simulink model "suspmod_yime_response"  (R2014a)
settings: Solver=ode45  SolverMode=SingleTasking  StartTime=0.0  StopTime=50  RelTol=1e-3  AbsTol=1e-6
settings Model: Creator=Rick  LastModifiedBy=JATIN
settings DataIOCC: LimitDataPoints=off  SignalLoggingSaveFormat=ModelDataLogs
settings OptimizationCC: BlockReduction=off  BooleanDataType=off  ExpressionDepthLimit=2147483647
settings DebuggingCC: SaveWithParameterizedLinksMsg=none  UnderspecifiedInitializationDetection=Classic  SignalResolutionControl=TryResolveAllWithWarning  SolverPrmCheckMsg=none  InheritedTsInSrcMsg=none  MultiTaskDSMMsg=warning  MultiTaskCondExecSysMsg=none  FcnCallInpInsideContextMsg=EnableAllAsWarning  UnknownTsInhSupMsg=none  StateNameClashWarn=warning
settings HardwareCC: TargetUnknown=on
settings RTWCC: IncludeERTFirstTime=on

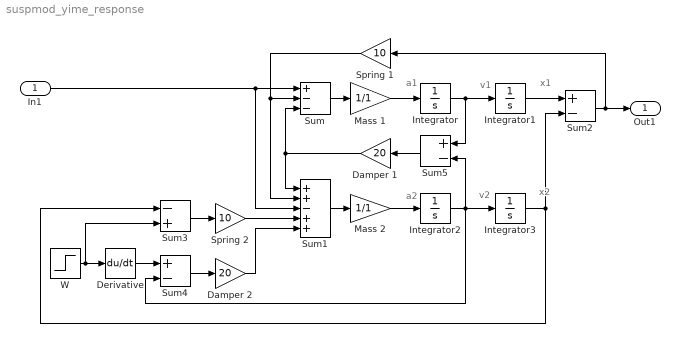
== system suspmod_yime_response ==
  note: a1
  note: v1
  note: x1
  note: a2
  note: v2
  note: x2
  In1 : Inport
  Damper 1 : Gain  Gain=20  SaturateOnIntegerOverflow=on  OutDataTypeStr=Inherit: Same as input  ParamDataTypeStr=Inherit: Same as input
  Damper 2 : Gain  Gain=20  SaturateOnIntegerOverflow=on  OutDataTypeStr=Inherit: Same as input  ParamDataTypeStr=Inherit: Same as input
  Derivative : Derivative
  Integrator{,1..3} (4 alike) : Integrator
  Mass 1 : Gain  Gain=1/1  SaturateOnIntegerOverflow=on  OutDataTypeStr=Inherit: Same as input  ParamDataTypeStr=Inherit: Same as input
  Mass 2 : Gain  Gain=1/1  SaturateOnIntegerOverflow=on  OutDataTypeStr=Inherit: Same as input  ParamDataTypeStr=Inherit: Same as input
  Spring 1 : Gain  Gain=10  SaturateOnIntegerOverflow=on  OutDataTypeStr=Inherit: Same as input  ParamDataTypeStr=Inherit: Same as input
  Spring 2 : Gain  Gain=10  SaturateOnIntegerOverflow=on  OutDataTypeStr=Inherit: Same as input  ParamDataTypeStr=Inherit: Same as input
  Sum : Sum  Inputs=+--  SaturateOnIntegerOverflow=on  InputSameDT=on  OutDataTypeStr=Inherit: Same as first input
  Sum1 : Sum  Inputs=++-++  SaturateOnIntegerOverflow=on  InputSameDT=on  OutDataTypeStr=Inherit: Same as first input
  Sum2 : Sum  Inputs=+-  SaturateOnIntegerOverflow=on  InputSameDT=on  OutDataTypeStr=Inherit: Same as first input
  Sum3 : Sum  Inputs=-+  SaturateOnIntegerOverflow=on  InputSameDT=on  OutDataTypeStr=Inherit: Same as first input
  Sum4 : Sum  Inputs=+-  SaturateOnIntegerOverflow=on  InputSameDT=on  OutDataTypeStr=Inherit: Same as first input
  Sum5 : Sum  Inputs=+-  SaturateOnIntegerOverflow=on  InputSameDT=on  OutDataTypeStr=Inherit: Same as first input
  W : Step  Time=0  After=0
  Out1 : Outport
  wires:
  Mass 2/1 -> Integrator2/1
  Sum1/1 -> Mass 2/1
  Integrator2/1 -> Integrator3/1, Sum4/2, Sum5/2
  Sum5/1 -> Damper 1/1
  Damper 1/1 -> Sum1/1, Sum/3
  Mass 1/1 -> Integrator/1
  Sum/1 -> Mass 1/1
  Integrator1/1 -> Sum2/1
  Integrator/1 -> Integrator1/1, Sum5/1
  Integrator3/1 -> Sum2/2, Sum3/1
  Sum2/1 -> Out1/1, Spring 1/1
  Spring 1/1 -> Sum/2, Sum1/2
  Damper 2/1 -> Sum1/5
  Spring 2/1 -> Sum1/4
  Sum3/1 -> Spring 2/1
  Sum4/1 -> Damper 2/1
  In1/1 -> Sum/1, Sum1/3
  Derivative/1 -> Sum4/1
  W/1 -> Sum3/2, Derivative/1
